simulink model "determineSimulationPhase_th"  (R2018a)
settings: Solver=FixedStepDiscrete  StartTime=0.0  StopTime=200  FixedStep=sm.Ts  RelTol=1e-3
libraries: determineIterationPhase_ul x1, determineSimulationPhase_ul x1, powerlib_meascontrol x1
settings Model: Creator=mitch  LastModifiedBy=mitch

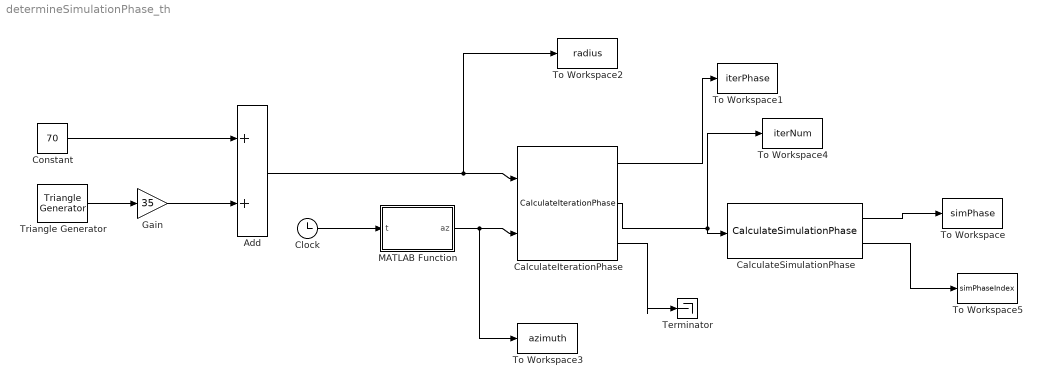
== system determineSimulationPhase_th ==
  Add : Sum
  CalculateIterationPhase : determineIterationPhase_ul/CalculateIterationPhase
  CalculateSimulationPhase : determineSimulationPhase_ul/CalculateSimulationPhase
      link override ResettableCounter/Constant: Value=0
  Clock : Clock
  Constant : Constant  Value=70
  Gain : Gain  Gain=35
  MATLAB Function : MATLAB Function  TreatAsAtomicUnit=on
  Terminator : Terminator
  To Workspace : ToWorkspace  VariableName=simPhase  SaveFormat=Timeseries  SampleTime=-1
  To Workspace1 : ToWorkspace  VariableName=iterPhase  SaveFormat=Timeseries  SampleTime=-1
  To Workspace2 : ToWorkspace  VariableName=radius  SaveFormat=Timeseries  SampleTime=-1
  To Workspace3 : ToWorkspace  VariableName=azimuth  SaveFormat=Timeseries  SampleTime=-1
  To Workspace4 : ToWorkspace  VariableName=iterNum  SaveFormat=Timeseries  SampleTime=-1
  To Workspace5 : ToWorkspace  VariableName=simPhaseIndex  SaveFormat=Timeseries  SampleTime=-1
  Triangle Generator : powerlib_meascontrol/Pulse & Signal Generators/Triangle Generator  Freq=0.1  Phase=90  Ts=0
  wires:
  CalculateSimulationPhase/1 -> To Workspace/1
  Clock/1 -> MATLAB Function/1(t)
  MATLAB Function/1(az) -> To Workspace3/1, CalculateIterationPhase/2
  Triangle Generator/1 -> Gain/1
  Constant/1 -> Add/1
  Gain/1 -> Add/2
  Add/1 -> To Workspace2/1, CalculateIterationPhase/1
  CalculateIterationPhase/2 -> To Workspace4/1, CalculateSimulationPhase/1
  CalculateIterationPhase/1 -> To Workspace1/1
  CalculateSimulationPhase/2 -> To Workspace5/1
  CalculateIterationPhase/3 -> Terminator/1

== matlab function determineSimulationPhase_th/MATLAB Function ==
  data: t input; az output
function az  = fcn(t)

az = sin(2*pi*t);
end
